simulink model "hw1_acc_model"  (Simulink 8.9)
settings: Solver=ode5  StartTime=0.0  StopTime=100  FixedStep=0.2  RelTol=1e-3  EnableMultiTasking=on
InitFcn:
  | m = 1000;
  | b = 50;
libraries: simulink x1
settings Model: Creator=kamesh  LastModifiedBy=edward
settings DataIOCC: FinalStateName=SimState  LimitDataPoints=off  MaxDataPoints=10  SaveCompleteFinalSimState=on
settings OptimizationCC: DefaultParameterBehavior=Inlined  UseFloatMulNetSlope=on  UseSpecifiedMinMax=on  InlineInvariantSignals=on  EnhancedBackFolding=on  ExpressionDepthLimit=2147483647  ZeroExternalMemoryAtStartup=off  ZeroInternalMemoryAtStartup=off  NoFixptDivByZeroProtection=on  EfficientFloat2IntCast=on  LifeSpan=1
settings HardwareCC: ProdBitPerInt=16  ProdBitPerPointer=16  ProdBitPerSizeT=16  ProdBitPerPtrDiffT=16  ProdIntDivRoundTo=Floor  ProdEndianess=BigEndian  ProdWordSize=16  ProdHWDeviceType=Freescale->HC(S)12
settings SFSimCC: MATLABDynamicMemAlloc=off
settings RTWCC: SystemTargetFile=ert.tlc  GenCodeOnly=on  TemplateMakefile=ert_default_tmf  PostCodeGenCommand=packNGo(buildInfo, {'packType' 'hierarchical'})  Description=Embedded Coder  GenerateReport=on  IncludeHyperlinkInReport=on  LaunchReport=on  GenerateCodeMetricsReport=on  RTWCompilerOptimization=on
settings CodeAppCC: IgnoreCustomStorageClasses=off  CustomSymbolStrType=$N$R$M  MATLABSourceComments=on  InternalIdentifier=Classic
settings ERTTargetCC: MultiwordLength=2048  GenerateSampleERTMain=on  InlinedParameterPlacement=NonHierarchical  ERTCustomFileTemplate=example_file_process.tlc  ConvertIfToSwitch=off  SuppressUnreachableDefaultCases=off

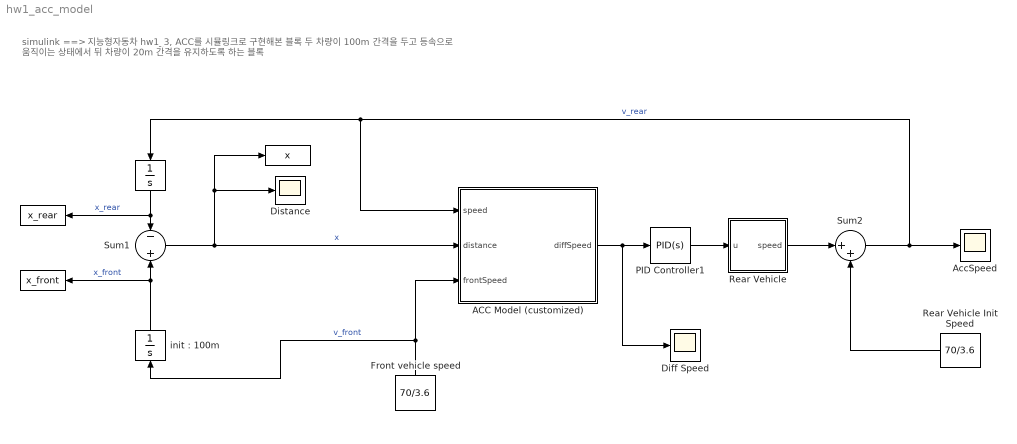
== system hw1_acc_model ==
  note: simulink ==> 지능형자동차 hw1_3, ACC를 시뮬링크로 구현해본 블록
      | 두 차량이 100m 간격을 두고 등속으로 움직이는 상태에서
      | 뒤 차량이 20m 간격을 유지하도록 하는 블록
  " " : Integrator
  "  " : ToWorkspace  VariableName=x_rear  SampleTime=-1
  "   " : ToWorkspace  VariableName=x_front  SampleTime=-1
  "      " : ToWorkspace  VariableName=x  SampleTime=-1
  ACC Model (customized) : Subsystem
  AccSpeed : Scope
  Diff Speed : Scope
  Distance : Scope
  Front vehicle speed : Constant  Value=70/3.6
  PID Controller1 : simulink/Continuous/PID Controller  Controller=PID  TimeDomain=Continuous-time  SampleTime=-1  IntegratorMethod=Forward Euler  FilterMethod=Forward Euler  Form=Parallel  UseFilter=on  ControllerParametersSource=internal  P=1000  I=120  D=0  N=100  InitialConditionSource=internal  InitialConditionForIntegrator=0  InitialConditionForFilter=0  ExternalReset=none  LimitOutput=off  UpperSaturationLimit=inf  LowerSaturationLimit=-inf  LinearizeAsGain=off  AntiWindupMode=none  Kb=1  TrackingMode=off  Kt=1  PParamMin=[]  PParamMax=[]  IParamMin=[]  IParamMax=[]  DParamMin=[]  DParamMax=[]  NParamMin=[]  NParamMax=[]  KbParamMin=[]  KbParamMax=[]  KtParamMin=[]  KtParamMax=[]  POutMin=[]  POutMax=[]  IOutMin=[]  IOutMax=[]  DOutMin=[]  DOutMax=[]  NOutMin=[]  NOutMax=[]  KbOutMin=[]  KbOutMax=[]  KtOutMin=[]  KtOutMax=[]  IntegratorOutMin=[]  IntegratorOutMax=[]  FilterOutMin=[]  FilterOutMax=[]  SumOutMin=[]  SumOutMax=[]  SumI1OutMin=[]  SumI1OutMax=[]  SumI2OutMin=[]  SumI2OutMax=[]  SumI3OutMin=[]  SumI3OutMax=[]  SumDOutMin=[]  SumDOutMax=[]  SaturationOutMin=[]  SaturationOutMax=[]  IntegratorContinuousStateAttributes=''  IntegratorStateMustResolveToSignalObject=off  IntegratorRTWStateStorageClass=Auto  FilterContinuousStateAttributes=''  FilterStateMustResolveToSignalObject=off  FilterRTWStateStorageClass=Auto  DifferentiatorICPrevScaledInput=0  DifferentiatorOutMin=[]  DifferentiatorOutMax=[]  InitialConditionSetting=State (most efficient)
  Rear Vehicle : Subsystem
  Rear Vehicle Init Speed : Constant  Value=70/3.6
  Sum1 : Sum  Inputs=-|+
  Sum2 : Sum  Inputs=|++
  "init : 100m" : Integrator  InitialCondition=100
  wires:
  ACC Model (customized)/1(diffSpeed) -> PID Controller1/1, Diff Speed/1
  Front vehicle speed/1 -> ACC Model (customized)/3(frontSpeed), "init : 100m"/1  "v_front"
  Sum1/1 -> ACC Model (customized)/2(distance), Distance/1, "      "/1  "x"
  PID Controller1/1 -> Rear Vehicle/1(u)
  Rear Vehicle Init Speed/1 -> Sum2/2
  Rear Vehicle/1(speed) -> Sum2/1
  Sum2/1 -> AccSpeed/1, ACC Model (customized)/1(speed), " "/1  "v_rear"
  "init : 100m"/1 -> Sum1/2, "   "/1  "x_front"
  " "/1 -> "  "/1, Sum1/1  "x_rear"

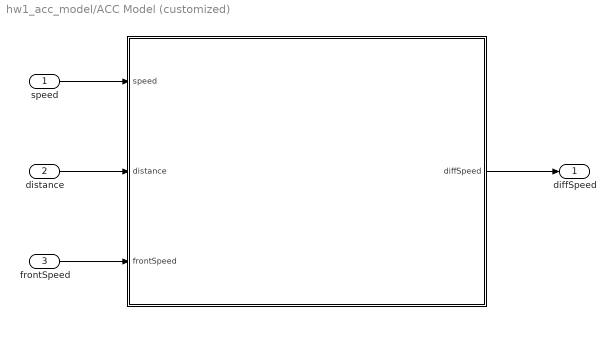
== system hw1_acc_model/ACC Model (customized) ==
  speed : Inport
  distance : Inport  Port=2
  frontSpeed : Inport  Port=3
  "          " : MATLAB Function  TreatAsAtomicUnit=on
  diffSpeed : Outport
  wires:
  distance/1 -> "          "/2(distance)
  "          "/1(diffSpeed) -> diffSpeed/1
  frontSpeed/1 -> "          "/3(frontSpeed)
  speed/1 -> "          "/1(speed)

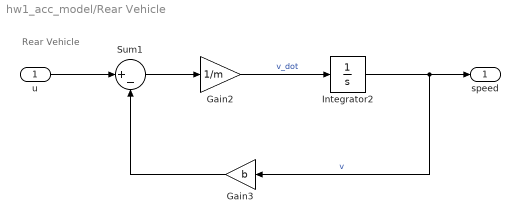
== system hw1_acc_model/Rear Vehicle ==
  note: Rear Vehicle
  u : Inport
  Gain2 : Gain  Gain=1/m
  Gain3 : Gain  Gain=b
  Integrator2 : Integrator
  Sum1 : Sum  Inputs=|+-
  speed : Outport
  wires:
  u/1 -> Sum1/1
  Integrator2/1 -> speed/1, Gain3/1  "v"
  Sum1/1 -> Gain2/1
  Gain2/1 -> Integrator2/1  "v_dot"
  Gain3/1 -> Sum1/2

== matlab function ACC Model (customized)/           ==
  data: speed input double; diffSpeed output double; distance input double; frontSpeed input double
function diffSpeed  = AccSubsystem(speed, distance, frontSpeed)

% dt와 a를 정한다
timeC=0.2;
acc_C = 8.5;

% 목표 거리
des_distance=20;

persistent setSpeed;

if isempty(setSpeed)
    setSpeed= 0;
end

minSpeed = 10;

% 등가속도 법칙에서 s = (vf^2 - vr^2) / 2a를 사용해서 rear vehicle이 dt동안 이동할 거리 구한다
% 너무 가까워지면 브레이크를 밟아야하므로 중요하다
deltaX=((frontSpeed*frontSpeed)-(speed*speed))/(2*(-acc_C));


% 실제거리가 des_distance보다 가까이 있는 경우
if(distance<=(des_distance + (deltaX)))
    if(distance <= deltaX + des_distance) && (distance  >= des_distance)
        tmpSpeed1 = sqrt((speed * speed) + (2*(-acc_C)*abs((deltaX + des_distance)-distance)));
        setSpeed = max(frontSpeed,tmpSpeed1);      % stops the reduction at front_speed.
        
    elseif(distance < des_distance)
        tmpSpeed2 = sqrt((speed * speed) + (2*(-acc_C)*abs(des_distance-distance)));
        setSpeed = max(minSpeed,tmpSpeed2);
    end

% 실제거리가 des_distane보다 멀리 있는 경우
elseif (distance>(des_distance + (deltaX)))
    setSpeed = speed + (acc_C * timeC);   % v = u + at
end

% 실제속도와 계산된 다음 속도의 차이를 반환합니다
diffSpeed = setSpeed - speed;
end
